simulink model "ports2"  (Simulink 8.3)
settings: Solver=ode45  StartTime=0.0  StopTime=10.0  RelTol=1e-3
settings Model: Creator=ladmin  LastModifiedBy=ladmin
settings DataIOCC: SignalLoggingSaveFormat=Dataset
settings DebuggingCC: UnderspecifiedInitializationDetection=Simplified  StateNameClashWarn=none
settings GRTTargetCC: CombineOutputUpdateFcns=on  GRTInterface=off

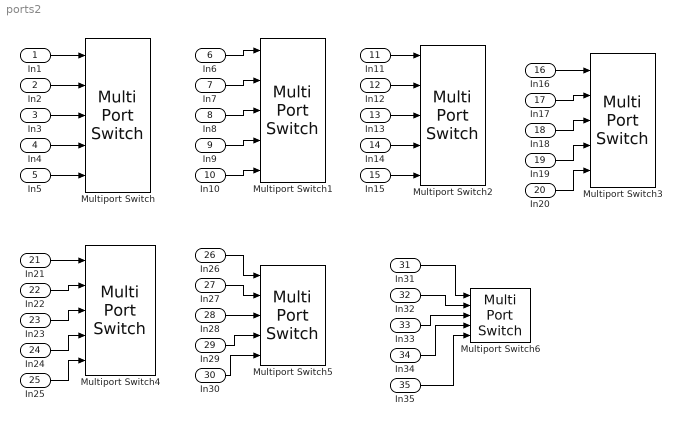
== system ports2 ==
  In1 : Inport
  In2 : Inport  Port=2
  In3 : Inport  Port=3
  In4 : Inport  Port=4
  In5 : Inport  Port=5
  In6 : Inport  Port=6
  In7 : Inport  Port=7
  In8 : Inport  Port=8
  In9 : Inport  Port=9
  In10 : Inport  Port=10
  In11 : Inport  Port=11
  In12 : Inport  Port=12
  In13 : Inport  Port=13
  In14 : Inport  Port=14
  In15 : Inport  Port=15
  In16 : Inport  Port=16
  In17 : Inport  Port=17
  In18 : Inport  Port=18
  In19 : Inport  Port=19
  In20 : Inport  Port=20
  In21 : Inport  Port=21
  In22 : Inport  Port=22
  In23 : Inport  Port=23
  In24 : Inport  Port=24
  In25 : Inport  Port=25
  In26 : Inport  Port=26
  In27 : Inport  Port=27
  In28 : Inport  Port=28
  In29 : Inport  Port=29
  In30 : Inport  Port=30
  In31 : Inport  Port=31
  In32 : Inport  Port=32
  In33 : Inport  Port=33
  In34 : Inport  Port=34
  In35 : Inport  Port=35
  Multiport Switch{,1..6} (7 alike) : MultiPortSwitch  Inputs=4
  wires:
  In5/1 -> Multiport Switch/5
  In4/1 -> Multiport Switch/4
  In3/1 -> Multiport Switch/3
  In2/1 -> Multiport Switch/2
  In1/1 -> Multiport Switch/1
  In10/1 -> Multiport Switch1/5
  In9/1 -> Multiport Switch1/4
  In8/1 -> Multiport Switch1/3
  In7/1 -> Multiport Switch1/2
  In6/1 -> Multiport Switch1/1
  In15/1 -> Multiport Switch2/5
  In14/1 -> Multiport Switch2/4
  In13/1 -> Multiport Switch2/3
  In12/1 -> Multiport Switch2/2
  In11/1 -> Multiport Switch2/1
  In20/1 -> Multiport Switch3/5
  In19/1 -> Multiport Switch3/4
  In18/1 -> Multiport Switch3/3
  In17/1 -> Multiport Switch3/2
  In16/1 -> Multiport Switch3/1
  In25/1 -> Multiport Switch4/5
  In24/1 -> Multiport Switch4/4
  In23/1 -> Multiport Switch4/3
  In22/1 -> Multiport Switch4/2
  In21/1 -> Multiport Switch4/1
  In30/1 -> Multiport Switch5/5
  In29/1 -> Multiport Switch5/4
  In28/1 -> Multiport Switch5/3
  In27/1 -> Multiport Switch5/2
  In26/1 -> Multiport Switch5/1
  In35/1 -> Multiport Switch6/5
  In34/1 -> Multiport Switch6/4
  In33/1 -> Multiport Switch6/3
  In32/1 -> Multiport Switch6/2
  In31/1 -> Multiport Switch6/1
